simulink model "LFC"  (R2024b)
settings: Solver=VariableStepAuto  StartTime=0.0  StopTime=30  RelTol=1e-3
values from neighbouring files (symbols this model uses):
  D = zeros(n,1)    [windcluster.m]
undefined symbols (not defined in the file or in its folder): FR, H, KIR, PFESS, RFESS, RR, t1, t2, TFESS, TR
settings Model: Creator=13103  LastModifiedBy=13103

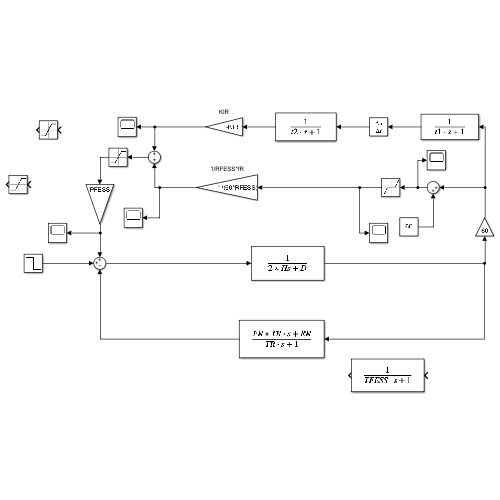
[thumbnail: Simulink's stored preview of the top-level diagram]
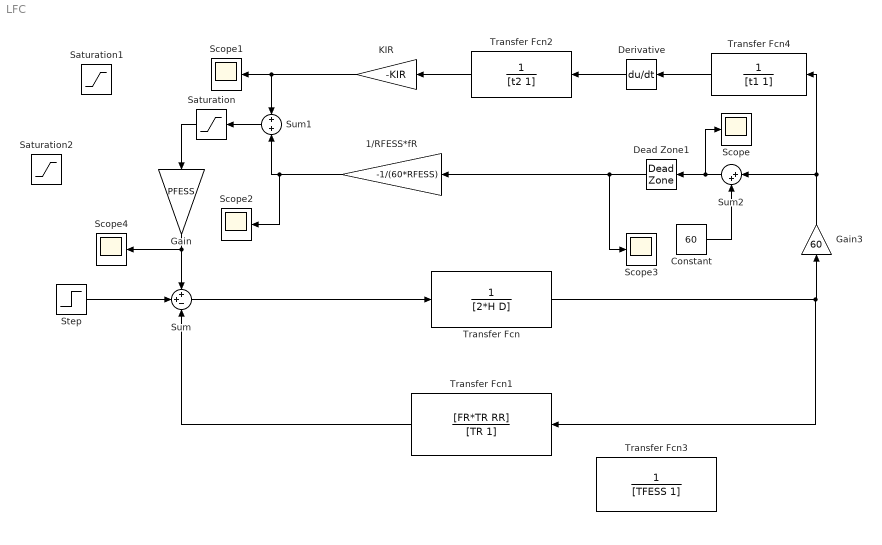
== system LFC ==
  1/RFESS*fR : Gain  Gain=-1/(60*RFESS)
  Constant : Constant  Value=60
  Dead Zone1 : DeadZone  LowerValue=59.6  UpperValue=60.4
  Derivative : Derivative
  Gain : Gain  Gain=PFESS
  Gain3 : Gain  Gain=60
  KIR : Gain  Gain=-KIR
  Saturation : Saturate  UpperLimit=1  LowerLimit=-1
  Saturation1 : Saturate  UpperLimit=1  LowerLimit=-1
  Saturation2 : Saturate  UpperLimit=1  LowerLimit=-1
  Scope{,1..4} (5 alike) : Scope
  Step : Step  Time=0  After=-7.55  SampleTime=0
  Sum : Sum  Inputs=++-
  Sum1 : Sum  Inputs=+|+
  Sum2 : Sum  Inputs=|++
  Transfer Fcn : TransferFcn  Denominator=[2*H D]
  Transfer Fcn1 : TransferFcn  Numerator=[FR*TR RR]  Denominator=[TR 1]
  Transfer Fcn2 : TransferFcn  Denominator=[t2 1]
  Transfer Fcn3 : TransferFcn  Denominator=[TFESS 1]
  Transfer Fcn4 : TransferFcn  Denominator=[t1 1]
  wires:
  Sum/1 -> Transfer Fcn/1
  Transfer Fcn/1 -> Transfer Fcn1/1, Gain3/1
  Step/1 -> Sum/2
  Saturation/1 -> Gain/1
  Transfer Fcn2/1 -> KIR/1
  Derivative/1 -> Transfer Fcn2/1
  Transfer Fcn4/1 -> Derivative/1
  Sum2/1 -> Dead Zone1/1, Scope/1
  Sum1/1 -> Saturation/1
  Gain3/1 -> Sum2/1, Transfer Fcn4/1
  Dead Zone1/1 -> 1/RFESS*fR/1, Scope3/1
  Constant/1 -> Sum2/2
  Transfer Fcn1/1 -> Sum/3
  KIR/1 -> Scope1/1, Sum1/1
  1/RFESS*fR/1 -> Sum1/2, Scope2/1
  Gain/1 -> Sum/1, Scope4/1
